simulink model "springDam"  (R2018b)
settings: Solver=VariableStepAuto  StartTime=0.0  StopTime=20  RelTol=1e-3
values from neighbouring files (symbols this model uses):
  m = 3    [mpctry.m]
undefined symbols (not defined in the file or in its folder): c, k
libraries: simulink x1
settings Model: Creator=nilay  LastModifiedBy=nilay

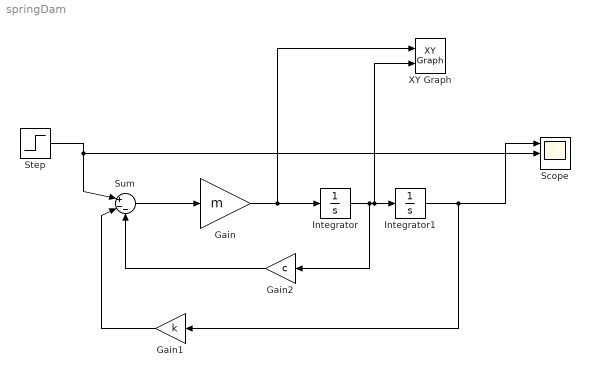
== system springDam ==
  Gain : Gain  Gain=m
  Gain1 : Gain  Gain=k
  Gain2 : Gain  Gain=c
  Integrator : Integrator
  Integrator1 : Integrator
  Scope : Scope  NumInputPorts=3
  Step : Step  SampleTime=0
  Sum : Sum  Inputs=|+--
  XY Graph : simulink/Sinks/XY Graph  xmin=-1  xmax=1  ymin=-1  ymax=1  st=-1
  wires:
  Integrator/1 -> Gain2/1, XY Graph/2, Integrator1/1
  Step/1 -> Scope/2, Sum/1
  Sum/1 -> Gain/1
  Gain/1 -> XY Graph/1, Integrator/1
  Integrator1/1 -> Scope/1, Gain1/1
  Gain1/1 -> Sum/2
  Gain2/1 -> Sum/3
